simulink model "ATABEY_Model_sim_old"  (R2025b)
settings: Solver=VariableStepAuto  StartTime=0.0  StopTime=simTime  RelTol=1e-3
InitFcn:
  | Trimhane
values from neighbouring files (symbols this model uses):
  chi_trim = 0    [Trimhane.m]
  eta_trim = 0.1    [Trimhane.m]
  fcPosRef = [100000 100000 1000]    [Trimhane.m]
  fcVelRef = [100 10 10]    [Trimhane.m]
  Kd_Ye = 0.6    [Trimhane.m]
  Kd_Ze = -0.05    [Trimhane.m]
  Ki_phi = -0.1    [Trimhane.m]
  Ki_psi = 0.001    [Trimhane.m]
  Ki_theta = -0.8    [Trimhane.m]
  Ki_u = 0.15    [Trimhane.m]
  Ki_Ye = 0.0025    [Trimhane.m]
  Ki_Ze = -0.0001    [Trimhane.m]
  Kp_phi = -0.2    [Trimhane.m]
  Kp_psi = 0.7    [Trimhane.m]
  Kp_theta = -0.8    [Trimhane.m]
  Kp_u = 0.5    [Trimhane.m]
  Kp_Xe = 0.125    [Trimhane.m]
  Kp_Ye = 0.18    [Trimhane.m]
  Kp_Ze = -0.3    [Trimhane.m]
  Kphi_xi = -0.2    [Trimhane.m]
  Kq_eta = -0.28    [Trimhane.m]
  Ktheta_eta = -1    [Trimhane.m]
  q_trim = 0    [Trimhane.m]
  tau_trim = 0    [Trimhane.m]
  theta_trim = 0    [Trimhane.m]
  UStar = [0.0259749326514 0.0259749326514 0.119240808134]    [ATABEY_trim_solution.mat]    (also in Trimhane.m = Z_star(10:12))
  xi_trim = 0    [Trimhane.m]
  XStar = [19.9815672328 -1.09212484719e-14 0.858470105267 7.6565722564e-16 1.89662146356e-14 -6.76749563554e-16 -1.43187171476e-15 0.0429366967763 -6.52464059676e-17]    [ATABEY_trim_solution.mat]    (also in Trimhane.m = Z_star(1:9))
libraries: aerolibfltsims x2, instrumentseriallib x2
settings Model: Creator=erayacikgz  LastModifiedBy=erayacikgz

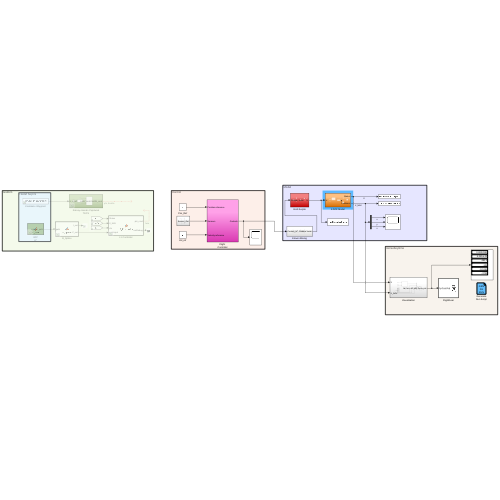
[thumbnail: Simulink's stored preview of the top-level diagram]
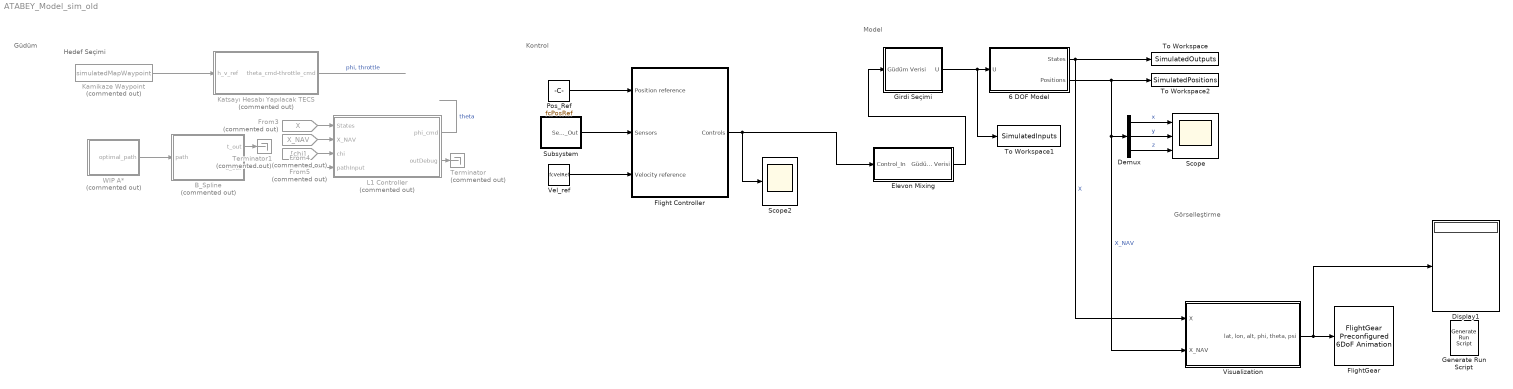
== system ATABEY_Model_sim_old ==
  note: Hedef Seçimi
  note: Görselleştirme
  note: Kontrol
  note: Güdüm
  note: Model
  6 DOF Model : Subsystem
  B_Spline : MATLAB Function  Commented=on  TreatAsAtomicUnit=on
  Demux : Demux  Outputs=3
  Display1 : Display
  Elevon Mixing : Subsystem
  Flight Controller : Subsystem
  "FlightGear " : aerolibfltsims/FlightGear Preconfigured 6DoF Animation  xFlightGearVersion=v2019.1  DestinationIpAddress=127.0.0.1  DestinationPort=5502  SampleTime=1/30  packetVersion=24
  From3 : From  Commented=on  GotoTag=X  TagVisibility=global
  From4 : From  Commented=on  GotoTag=X_NAV  TagVisibility=global
  From5 : From  Commented=on  GotoTag=chi  TagVisibility=global
  Generate Run Script : aerolibfltsims/Generate Run Script  Architecture=Linux  dataFlow=Send  GeometryModelName=c172p  AirportId=KSFO  RunwayId=10L  InitialAltitude=7224  InitialHeading=113  OffsetDistance=4.72  OffsetAzimuth=0  InstallScenery=off  DisableShaders=on  OriginAddress=127.0.0.1  DestinationPort=5502  OriginPort=5505  LocalAddress=127.0.0.1  OutputFileName=runfg.sh  FlightGearBaseDirectory=/usr/share/games/flightgear/
  Girdi Seçimi : Subsystem
  Kamikaze Waypoint : FromWorkspace  Commented=on  VariableName=simulatedMapWaypoint
  Katsayı Hesabı Yapılacak TECS : Subsystem  Commented=on
  L1 Controller : MATLAB Function  Commented=on  TreatAsAtomicUnit=on
  Pos_Ref : Constant  Value=fcPosRef
  Scope : Scope  NumInputPorts=3
      settings: ActiveDisplayYMinimum=-813.39775778773719  ActiveDisplayYMaximum=1636.3618951008921
  Scope2 : Scope
      settings: ActiveDisplayYMinimum=-5.0382411176791333  ActiveDisplayYMaximum=6.0841147965936591  DataLoggingVariableName=ScopeData2
  Subsystem : Subsystem
  Terminator : Terminator  Commented=on
  Terminator1 : Terminator  Commented=on
  To Workspace : ToWorkspace  VariableName=SimulatedOutputs  SaveFormat=Timeseries  SampleTime=-1
  To Workspace1 : ToWorkspace  VariableName=SimulatedInputs  SaveFormat=Timeseries  SampleTime=-1
  To Workspace2 : ToWorkspace  VariableName=SimulatedPositions  SaveFormat=Timeseries  SampleTime=-1
  Vel_ref : Constant  Value=fcVelRef
  Visualization : Subsystem
  WIP A* : MATLAB Function  Commented=on  TreatAsAtomicUnit=on
  wires:
  Elevon Mixing/1(Güdüm Verisi) -> Girdi Seçimi/1(Güdüm Verisi)
  6 DOF Model/2(Positions) -> To Workspace2/1, Demux/1, Visualization/2(X_NAV)  "X_NAV"
  6 DOF Model/1(States) -> To Workspace/1, Visualization/1(X)  "X"
  Demux/1 -> Scope/1  "x"
  Demux/2 -> Scope/2  "y"
  Demux/3 -> Scope/3  "z"
  Girdi Seçimi/1(U) -> To Workspace1/1, 6 DOF Model/1(U)
  Kamikaze Waypoint/1 -> Katsayı Hesabı Yapılacak TECS/1(h_v_ref)
  WIP A*/1(optimal_path) -> B_Spline/1(path)
  Pos_Ref/1 -> Flight Controller/1(Position reference)
  Vel_ref/1 -> Flight Controller/3(Velocity reference)
  Flight Controller/1(Controls) -> Elevon Mixing/1(Control_In), Scope2/1
  Subsystem/1(Sensor_Out) -> Flight Controller/2(Sensors)
  B_Spline/2(C_out) -> L1 Controller/4(pathInput)
  L1 Controller/2(outDebug) -> Terminator/1
  B_Spline/1(t_out) -> Terminator1/1
  From3/1 -> L1 Controller/1(States)
  From4/1 -> L1 Controller/2(X_NAV)
  From5/1 -> L1 Controller/3(chi)
  Visualization/1("lat, lon, alt, phi, theta, psi") -> Display1/1, "FlightGear "/1
  Katsayı Hesabı Yapılacak TECS/1(theta_cmd-throttle_cmd) -> ?  "phi, throttle"
  L1 Controller/1(phi_cmd) -> ?  "theta"

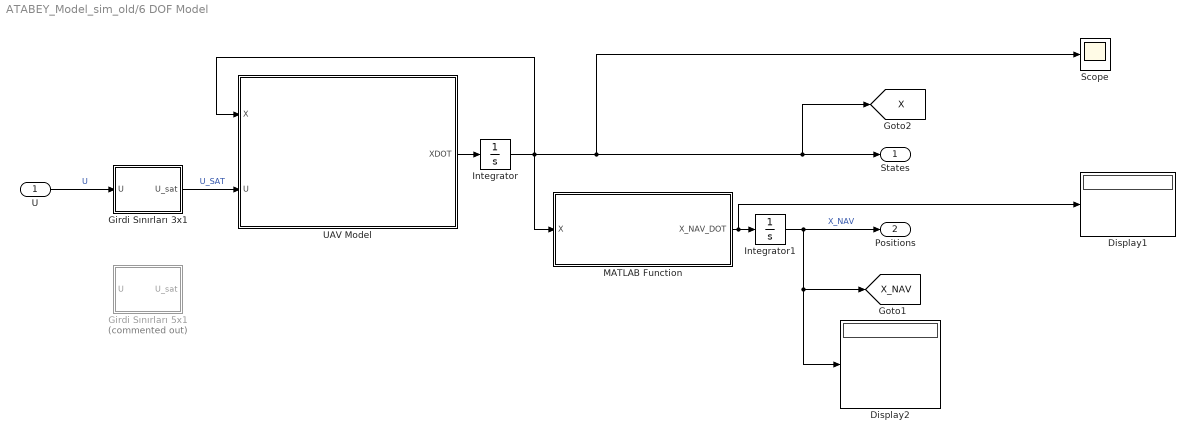
== system ATABEY_Model_sim_old/6 DOF Model ==
  U : Inport
  Display1 : Display
  Display2 : Display
  Girdi Sınırları 3x1 : Subsystem
  Girdi Sınırları 5x1 : Subsystem  Commented=on
  Integrator : Integrator  InitialCondition=XStar(:,:)
  Integrator1 : Integrator  InitialCondition=[0;0;1000;]
  MATLAB Function : MATLAB Function  TreatAsAtomicUnit=on
  Scope : Scope
      settings: ActiveDisplayYMinimum=-14.015843984237058  ActiveDisplayYMaximum=15.604004361685712
  UAV Model : MATLAB Function  TreatAsAtomicUnit=on
  States : Outport
  Positions : Outport  Port=2
  tag scope: X=global, X_NAV=global
  wires:
  Girdi Sınırları 3x1/1(U_sat) -> UAV Model/2(U)  "U_SAT"
  Integrator1/1 -> Display2/1, [X_NAV], Positions/1  "X_NAV"
  MATLAB Function/1(X_NAV_DOT) -> Display1/1, Integrator1/1
  Integrator/1 -> MATLAB Function/1(X), Scope/1, [X], States/1, UAV Model/1(X)
  UAV Model/1(XDOT) -> Integrator/1
  U/1 -> Girdi Sınırları 3x1/1(U)  "U"

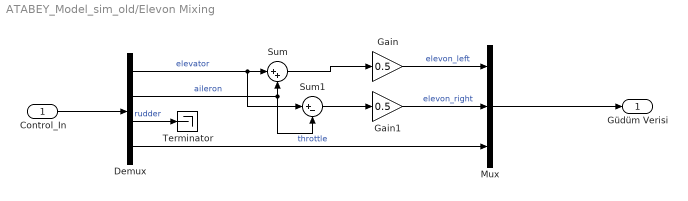
== system ATABEY_Model_sim_old/Elevon Mixing ==
  Control_In : Inport
  Demux : Demux
  Gain : Gain  Gain=0.5
  Gain1 : Gain  Gain=0.5
  Mux : Mux  Inputs=3
  Sum : Sum  Inputs=|++
  Sum1 : Sum  Inputs=|+-
  Terminator : Terminator
  Güdüm Verisi : Outport
  wires:
  Mux/1 -> Güdüm Verisi/1
  Control_In/1 -> Demux/1
  Demux/4 -> Mux/3  "throttle"
  Demux/3 -> Terminator/1  "rudder"
  Demux/2 -> Sum1/2, Sum/2  "aileron"
  Demux/1 -> Sum/1, Sum1/1  "elevator"
  Sum/1 -> Gain/1
  Sum1/1 -> Gain1/1
  Gain/1 -> Mux/1  "elevon_left"
  Gain1/1 -> Mux/2  "elevon_right"

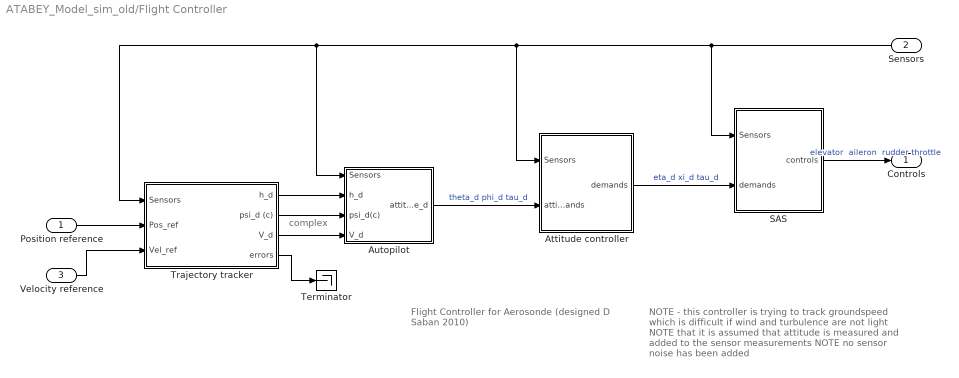
== system ATABEY_Model_sim_old/Flight Controller ==
  note: complex
  note: NOTE - this controller is trying to track
      | groundspeed which is difficult if wind
      | and turbulence are not light
      | NOTE that it is assumed that attitude is
      | measured and added to the sensor measurements
      | NOTE no sensor noise has been added
  note: Flight Controller
      | for Aerosonde
      | (designed D Saban 2010)
  Position reference : Inport
  Sensors : Inport  Port=2
  Velocity reference : Inport  Port=3
  Attitude controller : Subsystem
  Autopilot : Subsystem
  SAS : Subsystem
  Terminator : Terminator
  Trajectory tracker : Subsystem
  Controls : Outport
  wires:
  Trajectory tracker/3(V_d) -> Autopilot/4(V_d)
  Trajectory tracker/1(h_d) -> Autopilot/2(h_d)
  Trajectory tracker/4(errors) -> Terminator/1
  Velocity reference/1 -> Trajectory tracker/3(Vel_ref)
  Position reference/1 -> Trajectory tracker/2(Pos_ref)
  Trajectory tracker/2(psi_d (c)) -> Autopilot/3(psi_d(c))
  Autopilot/1(attitude_d) -> Attitude controller/2(attitude demands)  "theta_d phi_d tau_d"
  SAS/1(controls) -> Controls/1  "elevator  aileron  rudder throttle"
  Attitude controller/1(demands) -> SAS/2(demands)  "eta_d xi_d tau_d"
  Sensors/1 -> Trajectory tracker/1(Sensors), Autopilot/1(Sensors), Attitude controller/1(Sensors), SAS/1(Sensors)

== system ATABEY_Model_sim_old/Girdi Seçimi ==
  Güdüm Verisi : Inport
  Arduino RC Input : Subsystem  Commented=on
  Manual Switch : ManualSwitch  CurrentSetting=0
  Manual Switch1 : ManualSwitch  CurrentSetting=0
  Trim Input : Constant  Value=UStar(:,:)
  U : Outport
  wires:
  Güdüm Verisi/1 -> Manual Switch1/2
  Manual Switch/1 -> U/1  "U"
  Arduino RC Input/1(u_RC) -> Manual Switch1/1
  Manual Switch1/1 -> Manual Switch/2
  Trim Input/1 -> Manual Switch/1

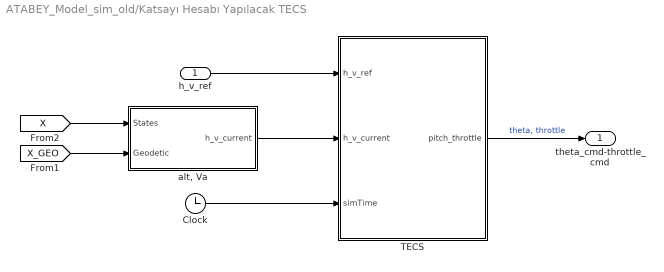
== system ATABEY_Model_sim_old/Katsayı Hesabı Yapılacak TECS ==
  h_v_ref : Inport
  Clock : Clock
  TECS : MATLAB Function  TreatAsAtomicUnit=on
  "alt, Va" : MATLAB Function  TreatAsAtomicUnit=on
  theta_cmd-throttle_cmd : Outport
  wires:
  h_v_ref/1 -> TECS/1(h_v_ref)
  Clock/1 -> TECS/3(simTime)
  "alt, Va"/1(h_v_current) -> TECS/2(h_v_current)
  TECS/1(pitch_throttle) -> theta_cmd-throttle_cmd/1  "theta, throttle"
  [X] -> "alt, Va"/1(States)
  [X_GEO] -> "alt, Va"/2(Geodetic)

== system ATABEY_Model_sim_old/Subsystem ==
  Demux1 : Demux  Outputs=[3 3 3]
  Mux : Mux  Inputs=[3 3 3 3]
  Sensor_Out : Outport
  wires:
  Demux1/1 -> Mux/2  "u v w"
  Demux1/3 -> Mux/4  "phi theta psi"
  Demux1/2 -> Mux/3  "p q r"
  [X_NAV] -> Mux/1  "P_N P_E h"
  [X] -> Demux1/1
  Mux/1 -> Sensor_Out/1

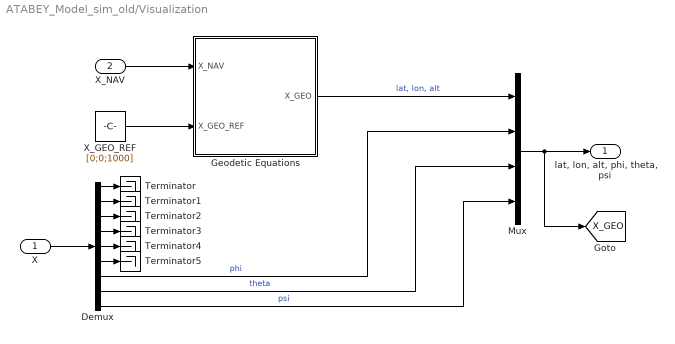
== system ATABEY_Model_sim_old/Visualization ==
  X : Inport
  X_NAV : Inport  Port=2
  Demux : Demux  Outputs=9
  Geodetic Equations : MATLAB Function  TreatAsAtomicUnit=on
  Mux : Mux
  Terminator{,1..5} (6 alike) : Terminator
  X_GEO_REF : Constant  Value=[0;0;1000]
  "lat, lon, alt, phi, theta, psi" : Outport
  tag scope: X_GEO=global
  wires:
  Mux/1 -> [X_GEO], "lat, lon, alt, phi, theta, psi"/1
  Geodetic Equations/1(X_GEO) -> Mux/1  "lat, lon, alt"
  Demux/9 -> Mux/4  "psi"
  Demux/7 -> Mux/2  "phi"
  X_NAV/1 -> Geodetic Equations/1(X_NAV)
  Demux/4 -> Terminator3/1
  X/1 -> Demux/1
  Demux/5 -> Terminator4/1
  X_GEO_REF/1 -> Geodetic Equations/2(X_GEO_REF)
  Demux/8 -> Mux/3  "theta"
  Demux/3 -> Terminator2/1
  Demux/2 -> Terminator1/1
  Demux/1 -> Terminator/1
  Demux/6 -> Terminator5/1

== system ATABEY_Model_sim_old/6 DOF Model/Girdi Sınırları 3x1 ==
  U : Inport
  Demux : Demux  Outputs=3
  Mux : Mux  Inputs=3
  Saturation : Saturate  UpperLimit=20  LowerLimit=-20
  Saturation1 : Saturate  UpperLimit=20  LowerLimit=-20
  Saturation3 : Saturate  UpperLimit=1  LowerLimit=0
  U_sat : Outport
  wires:
  Saturation3/1 -> Mux/3  "uThrottle_sat"
  Demux/3 -> Saturation3/1  "uThrottle"
  Saturation1/1 -> Mux/2  "uElevonRight_sat"
  Demux/1 -> Saturation/1  "uElevonLeft"
  Saturation/1 -> Mux/1  "uElevonLeft_sat"
  Demux/2 -> Saturation1/1  "uElevonRight"
  Mux/1 -> U_sat/1
  U/1 -> Demux/1

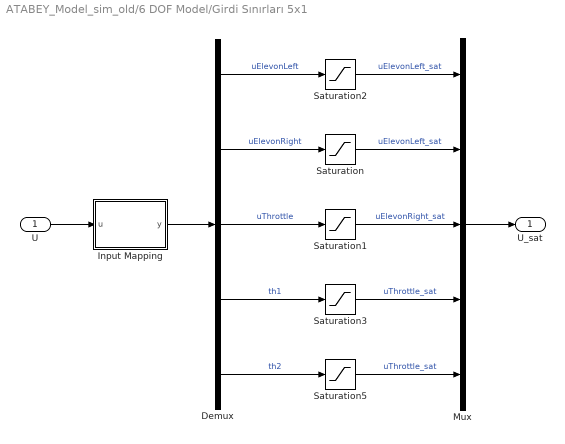
== system ATABEY_Model_sim_old/6 DOF Model/Girdi Sınırları 5x1 ==
  U : Inport
  Demux : Demux  Outputs=5
  Input Mapping : MATLAB Function  TreatAsAtomicUnit=on
  Mux : Mux  Inputs=5
  Saturation : Saturate  UpperLimit=20  LowerLimit=-20
  Saturation1 : Saturate  UpperLimit=20  LowerLimit=-20
  Saturation2 : Saturate  UpperLimit=20  LowerLimit=-20
  Saturation3 : Saturate  UpperLimit=1  LowerLimit=0
  Saturation5 : Saturate  UpperLimit=1  LowerLimit=0
  U_sat : Outport
  wires:
  U/1 -> Input Mapping/1(u)
  Mux/1 -> U_sat/1
  Input Mapping/1(y) -> Demux/1
  Demux/1 -> Saturation2/1  "uElevonLeft"
  Demux/2 -> Saturation/1  "uElevonRight"
  Demux/3 -> Saturation1/1  "uThrottle"
  Demux/4 -> Saturation3/1  "th1"
  Demux/5 -> Saturation5/1  "th2"
  Saturation2/1 -> Mux/1  "uElevonLeft_sat"
  Saturation/1 -> Mux/2  "uElevonLeft_sat"
  Saturation1/1 -> Mux/3  "uElevonRight_sat"
  Saturation3/1 -> Mux/4  "uThrottle_sat"
  Saturation5/1 -> Mux/5  "uThrottle_sat"

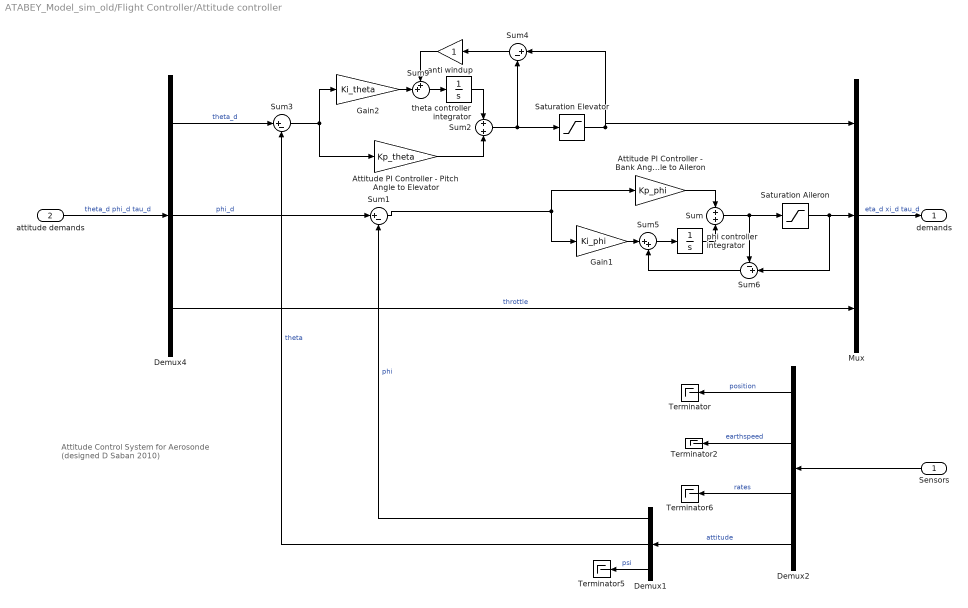
== system ATABEY_Model_sim_old/Flight Controller/Attitude controller ==
  note: Attitude Control System
      | for Aerosonde
      | (designed D Saban 2010)
  Sensors : Inport
  attitude demands : Inport  Port=2
  Attitude PI Controller - Bank Angle to Aileron : Gain  Gain=Kp_phi
  Attitude PI Controller - Pitch Angle to Elevator : Gain  Gain=Kp_theta
  Demux1 : Demux  Outputs=3
      settings: DisplayOption=none
  Demux2 : Demux  Outputs=[3 3 3 3]
  Demux4 : Demux  Outputs=3
      settings: DisplayOption=none
  Gain1 : Gain  Gain=Ki_phi
  Gain2 : Gain  Gain=Ki_theta
  Mux : Mux  Inputs=3
  Saturation Aileron : Saturate  UpperLimit=20*pi/180  LowerLimit=-20*pi/180  ZeroCross=off
  Saturation Elevator : Saturate  UpperLimit=20*pi/180  LowerLimit=-20*pi/180  ZeroCross=off
  Sum : Sum  Inputs=+|+
  Sum1 : Sum  Inputs=|+-
  Sum2 : Sum  Inputs=+|+
  Sum3 : Sum  Inputs=|+-
  Sum4 : Sum  Inputs=|+-
  Sum5 : Sum  Inputs=|++
  Sum6 : Sum  Inputs=-+|
  Sum9 : Sum  Inputs=++|
  Terminator{,2,5..6} (4 alike) : Terminator
  anti windup : Gain
  phi controller integrator : Integrator  InitialCondition=xi_trim
  theta controller integrator : Integrator  InitialCondition=eta_trim + Ktheta_eta*theta_trim + Kq_eta*q_trim
  demands : Outport
  wires:
  Sum6/1 -> Sum5/2
  Sum5/1 -> phi controller integrator/1
  Gain1/1 -> Sum5/1
  Saturation Aileron/1 -> Sum6/2, Mux/2
  Demux2/3 -> Terminator6/1  "rates"
  Demux1/3 -> Terminator5/1  "psi"
  Demux1/2 -> Sum3/2  "theta"
  Demux1/1 -> Sum1/2  "phi"
  Demux2/1 -> Terminator/1  "position"
  Sensors/1 -> Demux2/1
  Demux2/2 -> Terminator2/1  "earthspeed"
  Attitude PI Controller - Bank Angle to Aileron/1 -> Sum/1
  Demux4/1 -> Sum3/1  "theta_d"
  Mux/1 -> demands/1  "eta_d xi_d tau_d"
  attitude demands/1 -> Demux4/1  "theta_d phi_d tau_d"
  Demux4/3 -> Mux/3  "throttle"
  Sum/1 -> Sum6/1, Saturation Aileron/1
  phi controller integrator/1 -> Sum/2
  anti windup/1 -> Sum9/1
  Sum4/1 -> anti windup/1
  Saturation Elevator/1 -> Mux/1, Sum4/1
  Sum2/1 -> Sum4/2, Saturation Elevator/1
  Sum9/1 -> theta controller integrator/1
  Gain2/1 -> Sum9/2
  Attitude PI Controller - Pitch Angle to Elevator/1 -> Sum2/2
  theta controller integrator/1 -> Sum2/1
  Sum3/1 -> Attitude PI Controller - Pitch Angle to Elevator/1, Gain2/1
  Demux4/2 -> Sum1/1  "phi_d"
  Sum1/1 -> Gain1/1, Attitude PI Controller - Bank Angle to Aileron/1
  Demux2/4 -> Demux1/1  "attitude"

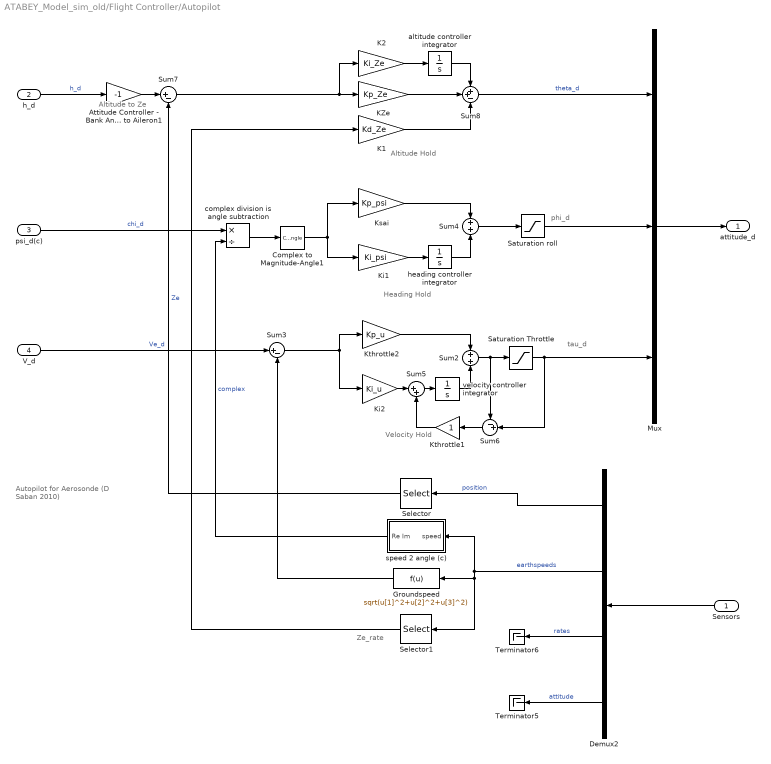
== system ATABEY_Model_sim_old/Flight Controller/Autopilot ==
  note: Autopilot
      | for Aerosonde
      | (D Saban 2010)
  note: Ze_rate
  note: tau_d
  note: phi_d
  note: Altitude Hold
  note: Velocity Hold
  note: Altitude to Ze
  note: Heading Hold
  Sensors : Inport
  h_d : Inport  Port=2
  psi_d(c) : Inport  Port=3
  V_d : Inport  Port=4
  Attitude Controller - Bank Angle to Aileron1 : Gain  Gain=-1
  Complex to Magnitude-Angle1 : ComplexToMagnitudeAngle  Output=Angle
  Demux2 : Demux  Outputs=[3 3 3 3]
  Groundspeed : Fcn  Expr=sqrt(u[1]^2+u[2]^2+u[3]^2)
  K1 : Gain  Gain=Kd_Ze
  K2 : Gain  Gain=Ki_Ze
  KZe : Gain  Gain=Kp_Ze
  Ki1 : Gain  Gain=Ki_psi
  Ki2 : Gain  Gain=Ki_u
  Ksai : Gain  Gain=Kp_psi
  Kthrottle1 : Gain
  Kthrottle2 : Gain  Gain=Kp_u
  Mux : Mux  Inputs=3
  Saturation Throttle : Saturate  UpperLimit=1  LowerLimit=0  ZeroCross=off
  Saturation roll : Saturate  UpperLimit=1.1  LowerLimit=-1.1  ZeroCross=off
  Selector : Selector  InputPortWidth=3  IndexOptions=Index vector (dialog)  Indices=3  OutputSizes=1
  Selector1 : Selector  InputPortWidth=3  IndexOptions=Index vector (dialog)  Indices=3  OutputSizes=1
  Sum2 : Sum
  Sum3 : Sum  Inputs=|+-
  Sum4 : Sum
  Sum5 : Sum  Inputs=|++
  Sum6 : Sum  Inputs=-+|
  Sum7 : Sum  Inputs=|+-
  Sum8 : Sum  Inputs=++-
  Terminator5 : Terminator
  Terminator6 : Terminator
  altitude controller integrator : Integrator  InitialCondition=theta_trim  LimitOutput=on  UpperSaturationLimit=.3  LowerSaturationLimit=-.3
  complex division is angle subtraction : Product  Inputs=*/
  heading controller integrator : Integrator  InitialCondition=chi_trim  LimitOutput=on  UpperSaturationLimit=1.2  LowerSaturationLimit=-1.2
  speed 2 angle (c) : Subsystem
  velocity controller integrator : Integrator  InitialCondition=tau_trim
  attitude_d : Outport
  wires:
  Complex to Magnitude-Angle1/1 -> Ki1/1, Ksai/1
  complex division is angle subtraction/1 -> Complex to Magnitude-Angle1/1
  speed 2 angle (c)/1(Re Im) -> complex division is angle subtraction/2  "complex"
  Saturation roll/1 -> Mux/2
  psi_d(c)/1 -> complex division is angle subtraction/1  "chi_d"
  Mux/1 -> attitude_d/1
  Selector1/1 -> K1/1
  heading controller integrator/1 -> Sum4/2
  Groundspeed/1 -> Sum3/2
  Selector/1 -> Sum7/2  "Ze"
  Demux2/4 -> Terminator5/1  "attitude"
  Demux2/3 -> Terminator6/1  "rates"
  Demux2/1 -> Selector/1  "position"
  Sensors/1 -> Demux2/1
  Demux2/2 -> speed 2 angle (c)/1(speed), Selector1/1, Groundspeed/1  "earthspeeds"
  Sum4/1 -> Saturation roll/1
  Sum8/1 -> Mux/1  "theta_d"
  V_d/1 -> Sum3/1  "Ve_d"
  h_d/1 -> Attitude Controller - Bank Angle to Aileron1/1  "h_d"
  Ki1/1 -> heading controller integrator/1
  Kthrottle1/1 -> Sum5/2
  Sum6/1 -> Kthrottle1/1
  velocity controller integrator/1 -> Sum2/2
  Sum5/1 -> velocity controller integrator/1
  Ki2/1 -> Sum5/1
  Saturation Throttle/1 -> Mux/3, Sum6/2
  Sum3/1 -> Ki2/1, Kthrottle2/1
  Sum2/1 -> Sum6/1, Saturation Throttle/1
  Kthrottle2/1 -> Sum2/1
  Attitude Controller - Bank Angle to Aileron1/1 -> Sum7/1
  K1/1 -> Sum8/3
  altitude controller integrator/1 -> Sum8/1
  K2/1 -> altitude controller integrator/1
  KZe/1 -> Sum8/2
  Sum7/1 -> K2/1, KZe/1
  Ksai/1 -> Sum4/1

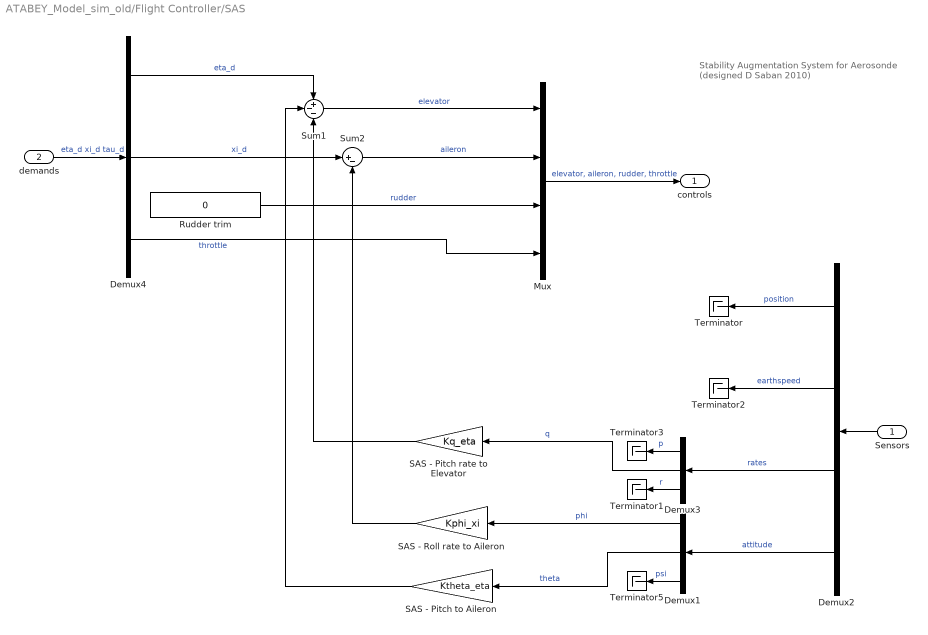
== system ATABEY_Model_sim_old/Flight Controller/SAS ==
  note: Stability Augmentation System
      | for Aerosonde
      | (designed D Saban 2010)
  Sensors : Inport
  demands : Inport  Port=2
  Demux1 : Demux  Outputs=3
      settings: DisplayOption=none
  Demux2 : Demux  Outputs=[3 3 3 3]
  Demux3 : Demux  Outputs=3
      settings: DisplayOption=none
  Demux4 : Demux  Outputs=3
      settings: DisplayOption=none
  Mux : Mux
  Rudder trim : Constant  Value=0
  SAS - Pitch rate to Elevator : Gain  Gain=Kq_eta
  SAS - Pitch to Aileron : Gain  Gain=Ktheta_eta
  SAS - Roll rate to Aileron : Gain  Gain=Kphi_xi
  Sum1 : Sum  Inputs=+--
  Sum2 : Sum  Inputs=|+-
  Terminator{,1..3,5} (5 alike) : Terminator
  controls : Outport
  wires:
  demands/1 -> Demux4/1  "eta_d xi_d tau_d"
  Mux/1 -> controls/1  "elevator, aileron, rudder, throttle"
  SAS - Pitch rate to Elevator/1 -> Sum1/3
  SAS - Roll rate to Aileron/1 -> Sum2/2
  Demux1/3 -> Terminator5/1  "psi"
  SAS - Pitch to Aileron/1 -> Sum1/2
  Demux1/2 -> SAS - Pitch to Aileron/1  "theta"
  Demux1/1 -> SAS - Roll rate to Aileron/1  "phi"
  Sum2/1 -> Mux/2  "aileron"
  Demux4/2 -> Sum2/1  "xi_d"
  Demux4/1 -> Sum1/1  "eta_d"
  Sum1/1 -> Mux/1  "elevator"
  Rudder trim/1 -> Mux/3  "rudder"
  Demux4/3 -> Mux/4  "throttle"
  Demux3/1 -> Terminator3/1  "p"
  Demux2/4 -> Demux1/1  "attitude"
  Demux2/1 -> Terminator/1  "position"
  Demux3/2 -> SAS - Pitch rate to Elevator/1  "q"
  Demux2/3 -> Demux3/1  "rates"
  Sensors/1 -> Demux2/1
  Demux2/2 -> Terminator2/1  "earthspeed"
  Demux3/3 -> Terminator1/1  "r"

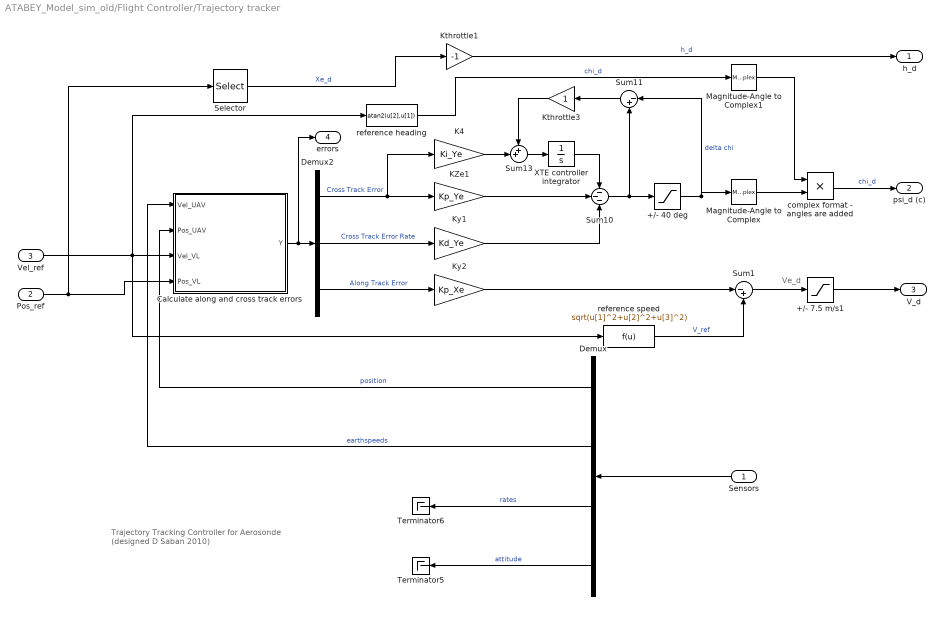
== system ATABEY_Model_sim_old/Flight Controller/Trajectory tracker ==
  note: Trajectory Tracking Controller
      | for Aerosonde
      | (designed D Saban 2010)
  note: Ve_d
  Sensors : Inport  PortDimensions=12
  Pos_ref : Inport  Port=2
  Vel_ref : Inport  Port=3
  +/- 40 deg : Saturate  UpperLimit=+40.0*pi/180  LowerLimit=-40*pi/180  ZeroCross=off
  +/- 7.5 m/s1 : Saturate  UpperLimit=90  LowerLimit=18  ZeroCross=off
  Calculate along and cross track errors : MATLAB Function  TreatAsAtomicUnit=on
  Demux : Demux  Outputs=[3 3 3 3]
  Demux2 : Demux  Outputs=3
  K4 : Gain  Gain=Ki_Ye
  KZe1 : Gain  Gain=Kp_Ye
  Kthrottle1 : Gain  Gain=-1
  Kthrottle3 : Gain
  Ky1 : Gain  Gain=Kd_Ye
  Ky2 : Gain  Gain=Kp_Xe
  Magnitude-Angle to Complex : MagnitudeAngleToComplex  Input=Angle  ConstantPart=1
  Magnitude-Angle to Complex1 : MagnitudeAngleToComplex  Input=Angle  ConstantPart=1
  Selector : Selector  InputPortWidth=3  IndexOptions=Index vector (dialog)  Indices=3  OutputSizes=1
  Sum1 : Sum  Inputs=|-+
  Sum10 : Sum  Inputs=---
  Sum11 : Sum  Inputs=|-+
  Sum13 : Sum  Inputs=++|
  Terminator5 : Terminator
  Terminator6 : Terminator
  XTE controller integrator : Integrator
  complex format - angles are added : Product  RndMeth=Zero
  reference heading : Fcn  Expr=atan2(u[2],u[1])
  reference speed : Fcn  Expr=sqrt(u[1]^2+u[2]^2+u[3]^2)
  h_d : Outport
  psi_d (c) : Outport  Port=2
  V_d : Outport  Port=3
  errors : Outport  Port=4
  wires:
  Magnitude-Angle to Complex1/1 -> complex format - angles are added/1
  Magnitude-Angle to Complex/1 -> complex format - angles are added/2
  reference heading/1 -> Magnitude-Angle to Complex1/1  "chi_d"
  +/- 40 deg/1 -> Magnitude-Angle to Complex/1, Sum11/1  "delta chi"
  complex format - angles are added/1 -> psi_d (c)/1  "chi_d"
  +/- 7.5 m/s1/1 -> V_d/1
  reference speed/1 -> Sum1/2  "V_ref"
  Sum1/1 -> +/- 7.5 m/s1/1
  Kthrottle1/1 -> h_d/1  "h_d"
  Selector/1 -> Kthrottle1/1  "Xe_d"
  Demux/4 -> Terminator5/1  "attitude"
  Demux/3 -> Terminator6/1  "rates"
  Demux/1 -> Calculate along and cross track errors/2(Pos_UAV)  "position"
  Sensors/1 -> Demux/1
  Demux/2 -> Calculate along and cross track errors/1(Vel_UAV)  "earthspeeds"
  Demux2/2 -> Ky1/1  "Cross Track Error Rate"
  Demux2/3 -> Ky2/1  "Along Track Error"
  Vel_ref/1 -> reference heading/1, reference speed/1, Calculate along and cross track errors/3(Vel_VL)
  Pos_ref/1 -> Selector/1, Calculate along and cross track errors/4(Pos_VL)
  Ky2/1 -> Sum1/1
  Calculate along and cross track errors/1(Y) -> errors/1, Demux2/1
  Demux2/1 -> K4/1, KZe1/1  "Cross Track Error"
  Ky1/1 -> Sum10/3
  Kthrottle3/1 -> Sum13/1
  Sum11/1 -> Kthrottle3/1
  Sum10/1 -> Sum11/2, +/- 40 deg/1
  XTE controller integrator/1 -> Sum10/1
  Sum13/1 -> XTE controller integrator/1
  K4/1 -> Sum13/2
  KZe1/1 -> Sum10/2

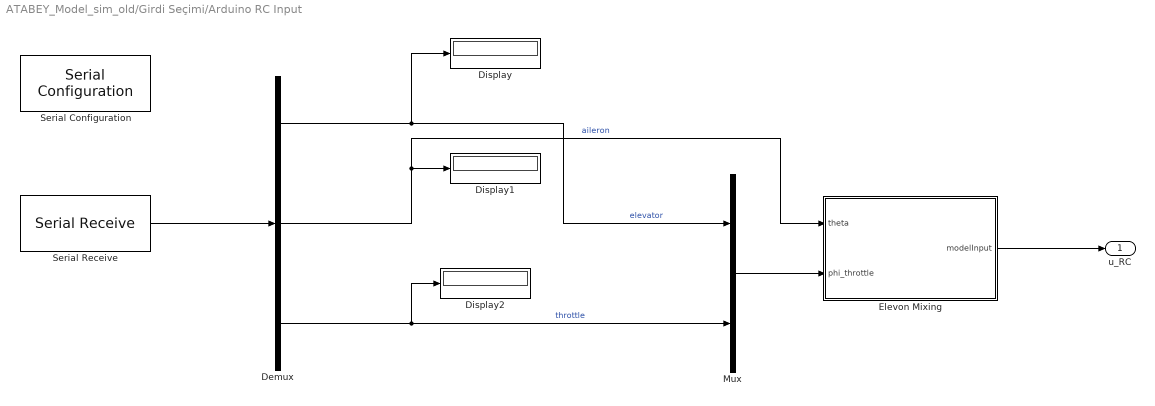
== system ATABEY_Model_sim_old/Girdi Seçimi/Arduino RC Input ==
  Demux : Demux  Outputs=3
  Display : Display
  Display1 : Display
  Display2 : Display
  Elevon Mixing : MATLAB Function  TreatAsAtomicUnit=on
  Mux : Mux  Inputs=2
  Serial Configuration : instrumentseriallib/Serial Configuration  Priority=-200000  PortSel=/dev/ttyUSB0  Port=/dev/ttyUSB0  ComPort=/dev/ttyUSB0  BaudRate=9600  DataBits=8  Parity=none  StopBits=1  ByteOrder=little-endian  FlowControl=none  Timeout=10  SimulateUsing=Interpreted execution  BlockInModel=on  aMode=1
      settings: LibrarySourceBlock=c2000lib/Host Communication/Serial Configuration
  Serial Receive : instrumentseriallib/Serial Receive  Priority=1  PortSel=/dev/ttyUSB0  Port=/dev/ttyUSB0  ComPort=/dev/ttyUSB0  DataType=int16  SaveDataType=uint8  ToggleHeader=on  Header=[255]  ToggleDataSize=on  DataSize=[1 3]  ToggleTerminator=off  Terminator=<none>  CustomTerminator=[]  InputFormat=Column major  EnableBlockingMode=on  ActionDataUnavailable=Output last received value  ActionWhenDataUnavailable=Output last received value  CustomValue=0  SampleTime=0.01  SimulateUsing=Interpreted execution  BlockInModel=on  aMode=1  LibraryInUse=c2000lib
      settings: LibrarySourceBlock=c2000lib/Host Communication/Serial Receive
  u_RC : Outport
  wires:
  Serial Receive/1 -> Demux/1
  Demux/3 -> Display2/1, Mux/2  "throttle"
  Demux/1 -> Mux/1, Display/1  "elevator"
  Demux/2 -> Elevon Mixing/1(theta), Display1/1  "aileron"
  Elevon Mixing/1(modelInput) -> u_RC/1
  Mux/1 -> Elevon Mixing/2(phi_throttle)

== system ATABEY_Model_sim_old/Flight Controller/Autopilot/speed 2 angle (c) ==
  speed : Inport
  Demux : Demux  Outputs=3
  Real-Imag to Complex : RealImagToComplex
  Terminator2 : Terminator
  Re Im : Outport
  wires:
  Demux/1 -> Real-Imag to Complex/1
  Demux/2 -> Real-Imag to Complex/2
  Demux/3 -> Terminator2/1
  Real-Imag to Complex/1 -> Re Im/1
  speed/1 -> Demux/1

== matlab function ATABEY_Model_sim_old/Katsayı Hesabı Yapılacak TECS/alt, Va ==
  data: States input; h_v_current output; Geodetic input
function h_v_current = fcn(States, Geodetic)

% Modelden ve Navigasyon Hesaplarından İrtifa ve Hız Çek

alt = Geodetic(3);

u = States(1); v = States(2); w = States(3);
Va = sqrt(u^2 + v^2 + w^2);

h_v_current = [alt,Va];

== matlab function ATABEY_Model_sim_old/6 DOF Model/MATLAB Function ==
  data: X input; X_NAV_DOT output
function X_NAV_DOT  = NavigationEquations(X)

P_N_dot = X(1)*cos(X(8))*cos(X(9))...
    + X(2)*(-cos(X(7))*sin(X(9)) + sin(X(7))*sin(X(8))*cos(X(9)))...
    + X(3)*(sin(X(7))*sin(X(9)) + cos(X(7))*sin(X(8))*cos(X(9)));

P_E_dot = X(1)*cos(X(8))*sin(X(9))...
    + X(2)*(cos(X(7))*cos(X(9)) + sin(X(7))*sin(X(8))*sin(X(9)))...
    + X(3)*(-sin(X(7))*cos(X(9)) + cos(X(7))*sin(X(8))*sin(X(9)));

h_dot = X(1)*sin(X(8)) - X(2)*sin(X(7))*cos(X(8)) - X(3)*cos(X(7))*cos(X(8));

X_NAV_DOT = [P_N_dot;
             P_E_dot;
             h_dot];

end

== matlab function ATABEY_Model_sim_old/6 DOF Model/UAV Model ==
  data: X input double size=[9 1]; XDOT output double size=[9 1]; U input double
% MATLAB/ATABEY_dynamics
% Fonksiyon, dinamik dosyasını çağırır, modüler değişiklik yapmak için

function XDOT = ATABEY_model(X, U)

    XDOT = ATABEY_dynamics(X, U);

end

== matlab function ATABEY_Model_sim_old/Visualization/Geodetic Equations ==
  data: X_NAV input; X_GEO output; X_GEO_REF input
function X_GEO = FlatEarthtoGeodetic(X_NAV, X_GEO_REF)

PN = X_NAV(1);               % Kuzey (m)
PE = X_NAV(2);               % Doğu  (m)
PH = X_NAV(3);               % Positive Down

lat0 = X_GEO_REF(1);
lon0 = X_GEO_REF(2);
alt0 = X_GEO_REF(3);

% WGS-84
a = 6378137.0;               % Semi-major axis (m)
f = 1/298.257223563;         % Flattening
e2 = 2*f - f^2;              % Eccentricity squared

lat0_rad = deg2rad(lat0);

% Eğri Yarıçapı, Prime Vertical
N = a / sqrt(1 - e2 * sin(lat0_rad)^2);

% Eğri Yarıçapı, Meridyen
M = a * (1 - e2) / (1 - e2 * sin(lat0_rad)^2)^1.5;

% PN/PE -> delta lat/lon (rad)
d_lat = PN / M;
d_lon = PE / (N * cos(lat0_rad));

% Çıktı
lat = lat0 + rad2deg(d_lat); % deg
lon = lon0 + rad2deg(d_lon); % deg
alt = alt0 - PH;             % m

X_GEO = [lat,lon,alt];

end

== matlab function ATABEY_Model_sim_old/WIP A* ==
  data: optimal_path output
function optimal_path = A_star()

    optimal_path = A_star();

end

== matlab function ATABEY_Model_sim_old/B_Spline ==
  data: t_out output; path input; C_out output
function [t_out, C_out] = B_Spline(path)

    [t_out, C_out] = B_Spline(path);

end

== matlab function ATABEY_Model_sim_old/L1 Controller ==
  data: States input; phi_cmd output; X_NAV input; chi input; outDebug output; pathInput input
function [phi_cmd, outDebug] = L1_Controller(States, X_NAV, chi, pathInput)

    [phi_cmd, outDebug] = L1_Controller(States, X_NAV, chi, pathInput);


end

== matlab function ATABEY_Model_sim_old/Katsayı Hesabı Yapılacak TECS/TECS ==
  data: h_v_ref input; h_v_current input; pitch_throttle output; simTime input
function pitch_throttle  = TECS( ...
    h_v_ref, ...                    % Referans irtifa (m), hız (m/s)
    h_v_current, ...                % Mevcut irtifa (m), hız (m/s)
    simTime)

%% GİRDİLER
mass = 2.5; g = 9.81;       % Araç kütlesi, yerçekimi ivmesi
Kp_E = 1; Ki_E = 1;         % Total Energy katsayılar
Kp_B = 1; Ki_B = 1;         % Energy Balance katsayılar

altitude_ref = h_v_ref(1); airspeed_ref = h_v_ref(2);
altitude_current = h_v_current(1); airspeed_current = h_v_current(2);

%% ENERJİ HESAPLARI

% Total Energy (E = mgh + 1/2 mV^2)
E     = mass * g * altitude_current + 0.5 * mass * airspeed_current^2;
E_ref = mass * g * altitude_ref + 0.5 * mass * airspeed_ref^2;
E_err = E_ref - E; % Energy error

% Energy Balance (Potansiyel ve kinetik enerji arasındaki fark)
B     = mass * g * altitude_current - 0.5 * mass * airspeed_current^2;
B_ref = mass * g * altitude_ref - 0.5 * mass * airspeed_ref^2;
B_err = B_ref - B; % Balance error

%% INTEGRAL HESABI
% Integralleri başlat
persistent int_E int_B
if isempty(int_E)
    int_E = 0;
end
if isempty(int_B)
    int_B = 0;
end

% Fonksiyon frekansını simülasyon frekansına eşitleme
persistent t_prev               
if isempty(t_prev)
    t_prev = simTime;
end

dt = simTime - t_prev;
t_prev = simTime;

int_E = int_E + E_err * dt;
int_B = int_B + B_err * dt;

%% PI KONTROL

% Throttle controls TOTAL ENERGY
throttle_cmd = Kp_E * E_err + Ki_E * int_E;

% Pitch controls ENERGY BALANCE
pitch_cmd = Kp_B * B_err + Ki_B * int_B;

%% SATURASYON
% Throttle (0-1)
throttle_cmd = min(max(throttle_cmd, 0), 1);

% Pitch (rad)
pitch_max = deg2rad(20);
pitch_cmd = min(max(pitch_cmd, -pitch_max), pitch_max);

pitch_throttle = [pitch_cmd throttle_cmd];

end

== matlab function ATABEY_Model_sim_old/Girdi Seçimi/Arduino RC Input/Elevon Mixing ==
  data: theta input; modelInput output; phi_throttle input
function modelInput  = elevonMix(theta, phi_throttle)
    phi = phi_throttle(1);
    
    % Elevon mixing
    elevon_left  = theta + phi;
    elevon_right = theta - phi;

    % % Clamp to actuator limits 
    % -> Gerek yok gibi?
    % elevon_left  = max(-1.0, min(1.0, elevon_left));
    % elevon_right = max(-1.0, min(1.0, elevon_right));

    % Throttle passthrough
    throttle_out = phi_throttle(2);

    modelInput = [elevon_left;elevon_right;throttle_out];

end

== matlab function ATABEY_Model_sim_old/6 DOF Model/Girdi Sınırları 5x1/Input Mapping ==
  data: u input; y output
function y = fcn(u)

% Map first two values from [-100, 100] to [-20, 20]
y1 = double(u(1)) * (20 / 100);
y2 = double(u(2)) * (20 / 100);

% Map last value from [0, 100] to [0, 1]
y3 = double(u(end)) * (1 / 100);

y = [y1; y2; y3];

== matlab function ATABEY_Model_sim_old/Flight Controller/Trajectory tracker/Calculate along and cross track errors ==
  data: Vel_UAV input; Pos_UAV input; Vel_VL input; Pos_VL input; Y output
function Y = track(Vel_UAV,Pos_UAV,Vel_VL,Pos_VL)

xVL = Pos_VL(1);
yVL = Pos_VL(2);
zVL = Pos_VL(3);

xUAV = Pos_UAV(1);
yUAV = Pos_UAV(2);
zUAV = Pos_UAV(3);

ChiVL = atan2(Vel_VL(2),Vel_VL(1));


% Distance between VL and UAV:
d_NED = [xUAV-xVL; yUAV-yVL; zUAV-zVL];

% Relative velocity between VL and UAV:
dV_NED = Vel_UAV - Vel_VL;

% Rotation matrix from NED to unD:
R = [cos(ChiVL) -sin(ChiVL) 0;
     sin(ChiVL)  cos(ChiVL) 0;
            0           0   1];

        
%----------------------------------------

d_unD = inv(R)*d_NED;
dV_unD = inv(R)*dV_NED;

ATD = d_unD(1);
OTD = d_unD(2);

dOTD = dV_unD(2);

%----------------------------------------

Y = [OTD; dOTD; ATD];
